simulink model "resonance_sin"  (R2022a)
settings: Solver=ode4  StartTime=0.0  StopTime=20  FixedStep=1e-3  MaxStep=1e-3  RelTol=1e-3
undefined symbols (not defined in the file): jsin
libraries: resonance_lib x1
settings Model: Creator=tstef  LastModifiedBy=tstef

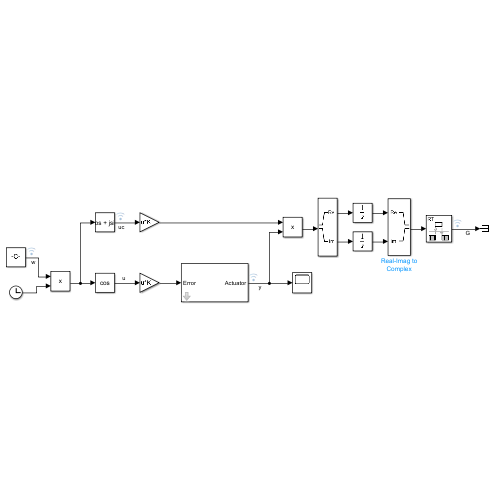
[thumbnail: Simulink's stored preview of the top-level diagram]
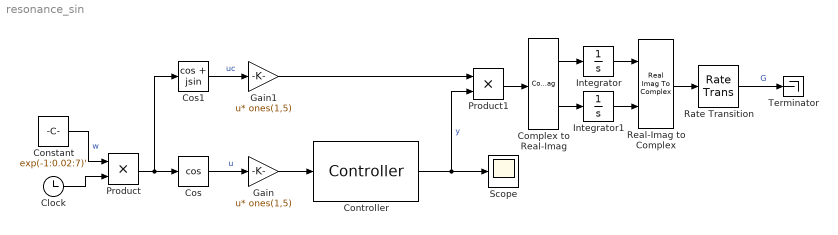
== system resonance_sin ==
  Clock : Clock
  Complex to Real-Imag : ComplexToRealImag
  Constant : Constant  Value=exp(-1:0.02:7)'  VectorParams1D=off
  Controller : resonance_lib/Controller  k_P=10  k_I=20  k_R=10  w0=100  zeta=0.05
  Cos : Trigonometry  Operator=cos
  Cos1 : Trigonometry  Operator=cos + jsin
  Gain : Gain  Gain=ones(1,5)  Multiplication=Matrix(u*K)
  Gain1 : Gain  Gain=ones(1,5)  Multiplication=Matrix(u*K)
  Integrator : Integrator
  Integrator1 : Integrator
  Product : Product
  Product1 : Product
  Rate Transition : RateTransition  Integrity=off  OutPortSampleTime=1
  Real-Imag to Complex : RealImagToComplex
  Scope : Scope
  Terminator : Terminator
  wires:
  Controller/1 -> Product1/2, Scope/1  "y"
  Gain/1 -> Controller/1
  Cos/1 -> Gain/1  "u"
  Constant/1 -> Product/1  "w"
  Clock/1 -> Product/2
  Product/1 -> Cos1/1, Cos/1
  Cos1/1 -> Gain1/1  "uc"
  Product1/1 -> Complex to Real-Imag/1
  Rate Transition/1 -> Terminator/1  "G"
  Gain1/1 -> Product1/1
  Complex to Real-Imag/1 -> Integrator/1
  Integrator/1 -> Real-Imag to Complex/1
  Integrator1/1 -> Real-Imag to Complex/2
  Complex to Real-Imag/2 -> Integrator1/1
  Real-Imag to Complex/1 -> Rate Transition/1
